simulink model "model_problems_16"  (R2021a)
settings: Solver=VariableStepAuto  StartTime=0.0  StopTime=10.0  RelTol=1e-3
model workspace (MAT data in the model file):
  K = 1
values from neighbouring files (symbols this model uses):
  feff = 2.4*10^-5    (= 2.4e-05)    [vars_problem_17_to_21.m]    (also in vars_problem_18_to_21.m; vars_problem_8_to_16.m)
  J_eff = [f(-f_11(x_11)), f(-f_22(x_22)),f(K4),f(2*K1)]    [vars_problem_17_to_21.m]    (also in vars_problem_18_to_21.m; vars_problem_8_to_16.m)
  K_D = [(2*Zeta*w_n*abs(J_eff(1))+1-feff)/kT,(2*Zeta*w_n*abs(J_eff(2))+1-feff)/kT,(2*Zeta*w_n*abs(J_eff(3))+1-feff)/kT,(2*Zeta*w_n*abs(J_eff(4))+1-feff)/kT]    [vars_problem_17_to_21.m]    (also in vars_problem_18_to_21.m; vars_problem_8_to_16.m)
  K_I = [w_n^2/kT,w_n^2/kT,w_n^2/kT,w_n^2/kT]    [vars_problem_17_to_21.m]    (also in vars_problem_18_to_21.m; vars_problem_8_to_16.m)
  K_P = [(2*Zeta*w_n+w_n^2*abs(J_eff(1)))/kT,(2*Zeta*w_n+w_n^2*abs(J_eff(2)))/kT,(2*Zeta*w_n+w_n^2*abs(J_eff(3)))/kT,(2*Zeta*w_n+w_n^2*abs(J_eff(4)))/kT]    [vars_problem_17_to_21.m]    (also in vars_problem_18_to_21.m; vars_problem_8_to_16.m)
  kT = 0.17    [vars_problem_17_to_21.m]    (also in vars_problem_18_to_21.m; vars_problem_8_to_16.m)
  ni = 53    [vars_problem_17_to_21.m]    (also in vars_problem_18_to_21.m; vars_problem_8_to_16.m)
  q_r = 0.35    [vars_problem_17_to_21.m]    (also in vars_problem_18_to_21.m; vars_problem_8_to_16.m)
  Tl = [0 fhq_2(q_max) fhq_3(q_max) fhq_4(q_max)]    [vars_problem_17_to_21.m]    (also in vars_problem_18_to_21.m; vars_problem_8_to_16.m)
settings Model: Creator=simon  LastModifiedBy=simon

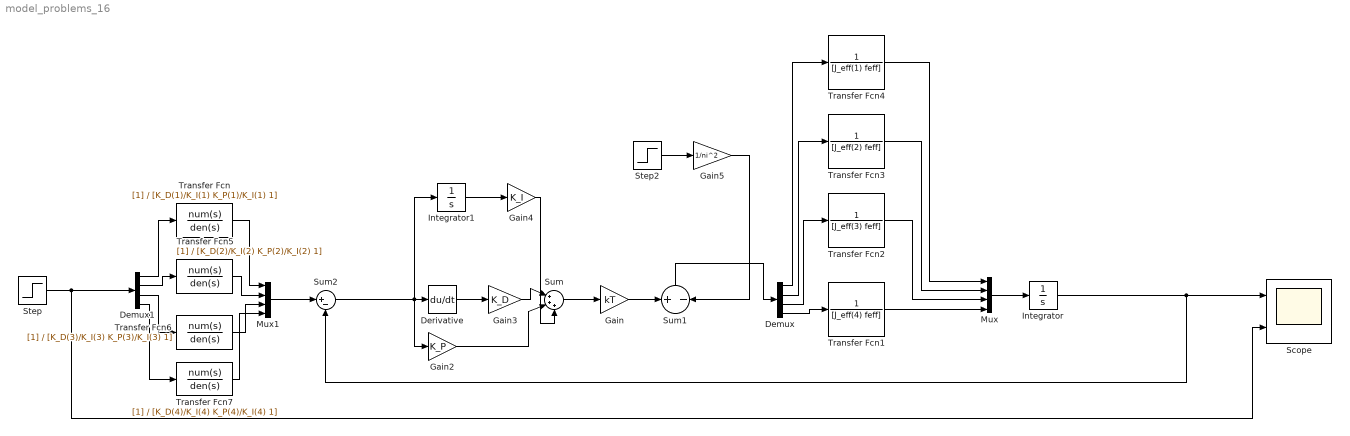
== system model_problems_16 ==
  Demux : Demux
  Demux1 : Demux
  Derivative : Derivative
  Gain : Gain  Gain=kT
  Gain2 : Gain  Gain=K_P
  Gain3 : Gain  Gain=K_D
  Gain4 : Gain  Gain=K_I
  Gain5 : Gain  Gain=1/ni^2
  Integrator : Integrator
  Integrator1 : Integrator
  Mux : Mux
  Mux1 : Mux
  Scope : Scope  NumInputPorts=2
  Step : Step  After=[q_r q_r q_r q_r]
  Step2 : Step  After=Tl  SampleTime=0
  Sum : Sum  Inputs=|+++
  Sum1 : Sum  Inputs=+-
  Sum2 : Sum  Inputs=|+-
  Transfer Fcn : TransferFcn  Denominator=[K_D(1)/K_I(1) K_P(1)/K_I(1) 1]
  Transfer Fcn1 : TransferFcn  Denominator=[J_eff(4) feff]
  Transfer Fcn2 : TransferFcn  Denominator=[J_eff(3) feff]
  Transfer Fcn3 : TransferFcn  Denominator=[J_eff(2) feff]
  Transfer Fcn4 : TransferFcn  Denominator=[J_eff(1) feff]
  Transfer Fcn5 : TransferFcn  Denominator=[K_D(2)/K_I(2) K_P(2)/K_I(2) 1]
  Transfer Fcn6 : TransferFcn  Denominator=[K_D(3)/K_I(3) K_P(3)/K_I(3) 1]
  Transfer Fcn7 : TransferFcn  Denominator=[K_D(4)/K_I(4) K_P(4)/K_I(4) 1]
  wires:
  Integrator/1 -> Scope/1, Sum2/2
  Gain/1 -> Sum1/1
  Step/1 -> Scope/2, Demux1/1
  Sum1/1 -> Demux/1
  Transfer Fcn1/1 -> Mux/4
  Transfer Fcn2/1 -> Mux/3
  Transfer Fcn3/1 -> Mux/2
  Transfer Fcn4/1 -> Mux/1
  Mux/1 -> Integrator/1
  Demux/1 -> Transfer Fcn4/1
  Demux/2 -> Transfer Fcn3/1
  Demux/3 -> Transfer Fcn2/1
  Demux/4 -> Transfer Fcn1/1
  Gain2/1 -> Sum/2
  Sum/1 -> Gain/1
  Sum2/1 -> Integrator1/1, Gain2/1, Derivative/1
  Gain3/1 -> Sum/1
  Derivative/1 -> Gain3/1
  Integrator1/1 -> Gain4/1
  Gain4/1 -> Sum/3
  Demux1/1 -> Transfer Fcn/1
  Demux1/2 -> Transfer Fcn5/1
  Demux1/3 -> Transfer Fcn6/1
  Demux1/4 -> Transfer Fcn7/1
  Transfer Fcn/1 -> Mux1/1
  Transfer Fcn5/1 -> Mux1/2
  Transfer Fcn6/1 -> Mux1/3
  Transfer Fcn7/1 -> Mux1/4
  Gain5/1 -> Sum1/2
  Step2/1 -> Gain5/1
  Mux1/1 -> Sum2/1
